simulink model "bungee"  (Simulink 7.4)
settings: Solver=ode45  StartTime=0.0  StopTime=100  MaxStep=0.1  RelTol=1e-3
values from neighbouring files (symbols this model uses):
  a1 = 1    [bungee_param.m]    (also in bungeescript.m)
  a2 = 1    [bungee_param.m]    (also in bungeescript.m)
  k = 5    [bungee_param.m]    (also in find_edge.m = ( y1 == min(y1) ); find_edge1.m = ( y1 == min(y1) ); find_edge2.m = ( y1 == min(y1) ); main_persistent.m = i - 1)
  m = 90    [bungee_param.m]    (also in bungeescript.m; main_bicycle1.m = 2045)
settings Model: Creator=user  LastModifiedBy=user
settings OptimizationCC: InitFltsAndDblsToZero=on
settings DebuggingCC: SaveWithParameterizedLinksMsg=none  SignalResolutionControl=TryResolveAllWithWarning  MultiTaskDSMMsg=warning  MultiTaskCondExecSysMsg=none
settings RTWCC: IncludeERTFirstTime=on
settings GRTTargetCC: TargetFcnLib=ansi_tfl_tmw.mat

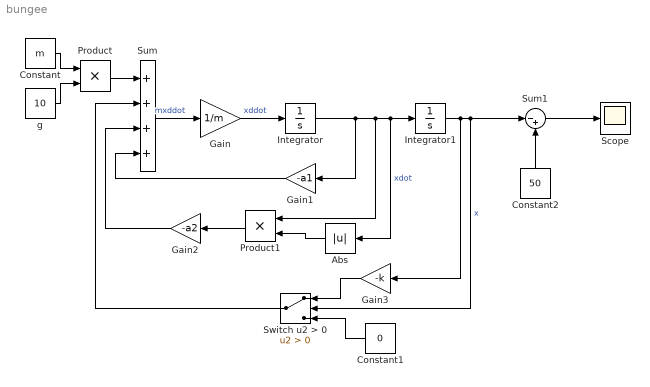
== system bungee ==
  Abs : Abs
  Constant : Constant  Value=m  OutDataType=sfix(16)  OutScaling=2^0
  Constant1 : Constant  Value=0  OutDataType=sfix(16)  OutScaling=2^0
  Constant2 : Constant  Value=50  OutDataType=sfix(16)  OutScaling=2^0
  Gain : Gain  Gain=1/m  ParameterDataType=sfix(16)  ParameterScaling=2^0  OutDataType=sfix(16)  OutScaling=2^0
  Gain1 : Gain  Gain=-a1  ParameterDataType=sfix(16)  ParameterScaling=2^0  OutDataType=sfix(16)  OutScaling=2^0
  Gain2 : Gain  Gain=-a2  ParameterDataType=sfix(16)  ParameterScaling=2^0  OutDataType=sfix(16)  OutScaling=2^0
  Gain3 : Gain  Gain=-k  ParameterDataType=sfix(16)  ParameterScaling=2^0  OutDataType=sfix(16)  OutScaling=2^0
  Integrator : Integrator
  Integrator1 : Integrator  InitialCondition=-30
  Product : Product  OutDataType=sfix(16)  OutScaling=2^0  RndMeth=Zero
  Product1 : Product  OutDataType=sfix(16)  OutScaling=2^0  RndMeth=Zero
  Scope : Scope
  Sum : Sum  Inputs=++++  OutDataType=sfix(16)  OutScaling=2^0
  Sum1 : Sum  Inputs=|-+  OutDataType=sfix(16)  OutScaling=2^0
  Switch u2 > 0 : Switch  Criteria=u2 > Threshold
  g : Constant  Value=10  OutDataType=sfix(16)  OutScaling=2^0
  wires:
  Constant/1 -> Product/1
  g/1 -> Product/2
  Product/1 -> Sum/1
  Sum/1 -> Gain/1  "mxddot"
  Gain/1 -> Integrator/1  "xddot"
  Integrator/1 -> Gain1/1, Product1/1, Integrator1/1, Abs/1  "xdot"
  Integrator1/1 -> Gain3/1, Switch u2 > 0/2, Sum1/1  "x"
  Gain1/1 -> Sum/4
  Product1/1 -> Gain2/1
  Abs/1 -> Product1/2
  Gain2/1 -> Sum/3
  Gain3/1 -> Switch u2 > 0/1
  Constant1/1 -> Switch u2 > 0/3
  Switch u2 > 0/1 -> Sum/2
  Constant2/1 -> Sum1/2
  Sum1/1 -> Scope/1
